simulink model "chirp1"  (Simulink 4.00)
settings: Solver=ode45  StartTime=0.0  StopTime=10.0  RelTol=1e-3
values from neighbouring files (symbols this model uses):
  delta_f = 2e3    (= 2000)    [chirp_1.m]    (also in fmasse_var_1.m = 0.390625; fmasse_var_2.m = 0.390625)
  f0 = 500    [chirp_1.m]    (also in costas1f.m = pf0; op_freq.m = 15; pll_5f.m = f01)
  T = 10e-3    (= 0.01)    [chirp_1.m]
libraries: simulink3 x1
settings Model: LastModifiedBy=Administrator  LimitDataPoints=off  BlockReductionOpt=off

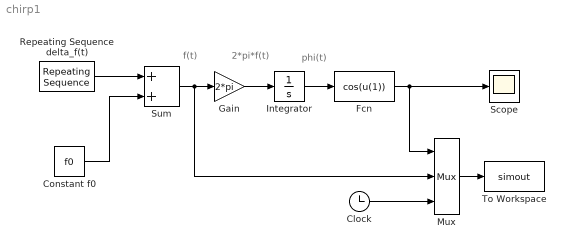
== system chirp1 ==
  note: f(t)
  note: 2*pi*f(t)
  note: phi(t)
  Clock : Clock
      settings: DisplayTime=off  Decimation=10
  Constant f0 : Constant  Value=f0
  Fcn : Fcn  Expr=cos(u(1))
  Gain : Gain  Gain=2*pi  Multiplication=Element-wise(K.*u)  SaturateOnIntegerOverflow=on
  Integrator : Integrator  ExternalReset=none  InitialConditionSource=internal  InitialCondition=0  LimitOutput=off  UpperSaturationLimit=inf  LowerSaturationLimit=-inf  ShowSaturationPort=off  ShowStatePort=off  AbsoluteTolerance=auto
  Mux : Mux  Inputs=3
      settings: DisplayOption=none
  Repeating Sequence delta_f(t) : simulink3/Sources/Repeating Sequence  rep_seq_t=[0 T 2*T]  rep_seq_y=[0 delta_f 0]
  Scope : Scope
      settings: TimeRange=auto  YMin=-5  YMax=5  SaveToWorkspace=off  SaveName=ScopeData  LimitDataPoints=on  MaxDataPoints=5000
  Sum : Sum  Inputs=++  SaturateOnIntegerOverflow=on
  To Workspace : ToWorkspace  VariableName=simout  SampleTime=-1  SaveFormat=Array
  wires:
  Repeating Sequence delta_f(t)/1 -> Sum/1
  Constant f0/1 -> Sum/2
  Sum/1 -> Gain/1, Mux/2
  Gain/1 -> Integrator/1
  Integrator/1 -> Fcn/1
  Fcn/1 -> Scope/1, Mux/1
  Mux/1 -> To Workspace/1
  Clock/1 -> Mux/3
